simulink model "trail"  (R2023b)
settings: Solver=VariableStepAuto  StartTime=0.0  StopTime=10.0  RelTol=1e-3
settings Model: Creator=Ahmed Raamadan  LastModifiedBy=Ahmed Raamadan

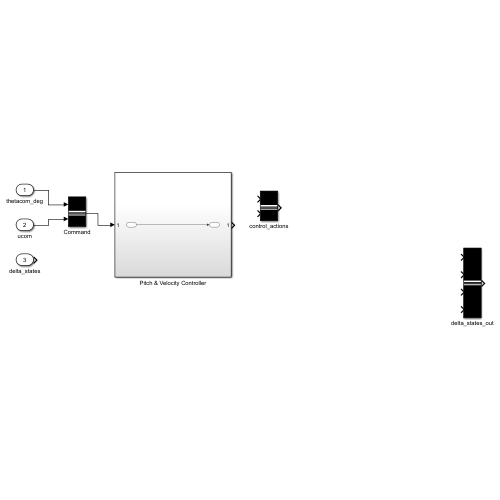
[thumbnail: Simulink's stored preview of the top-level diagram]
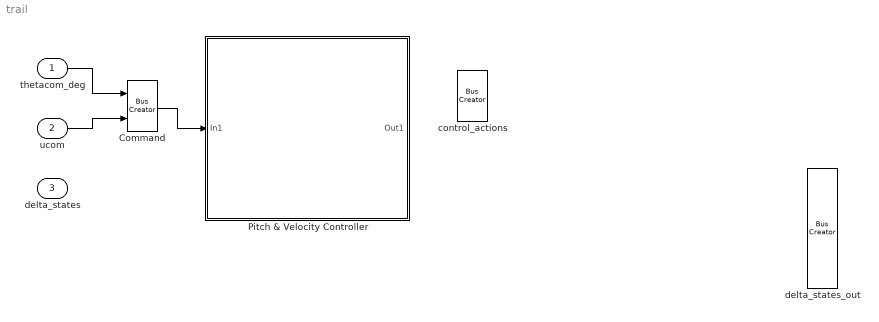
== system trail ==
  thetacom_deg : Inport
  ucom : Inport  Port=2
  delta_states : Inport  Port=3
  Command : BusCreator  Inputs=2
  Pitch & Velocity Controller : Subsystem
  control_actions : BusCreator  Inputs=2
  delta_states_out : BusCreator  Inputs=4
  wires:
  thetacom_deg/1 -> Command/1
  ucom/1 -> Command/2
  Command/1 -> Pitch & Velocity Controller/1(In1)

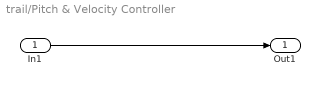
== system trail/Pitch & Velocity Controller ==
  In1 : Inport
  Out1 : Outport
  wires:
  In1/1 -> Out1/1
